simulink model "AA136_Sim"  (R2023b)
settings: Solver=VariableStepAuto  StartTime=0.0  StopTime=500  RelTol=1e-3
libraries: raspberrypiBasiclib x6
settings Model: Creator=ANWILEY-GREEN  LastModifiedBy=reedv

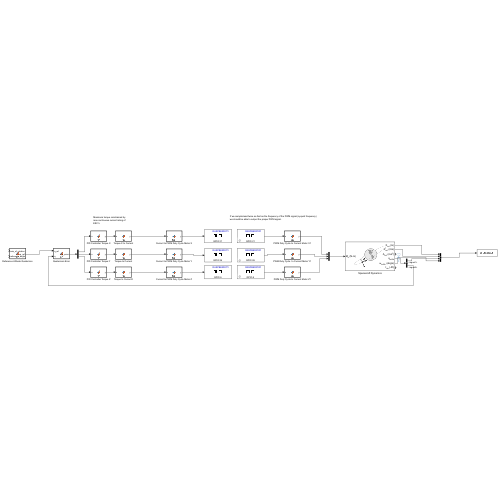
[thumbnail: Simulink's stored preview of the top-level diagram]
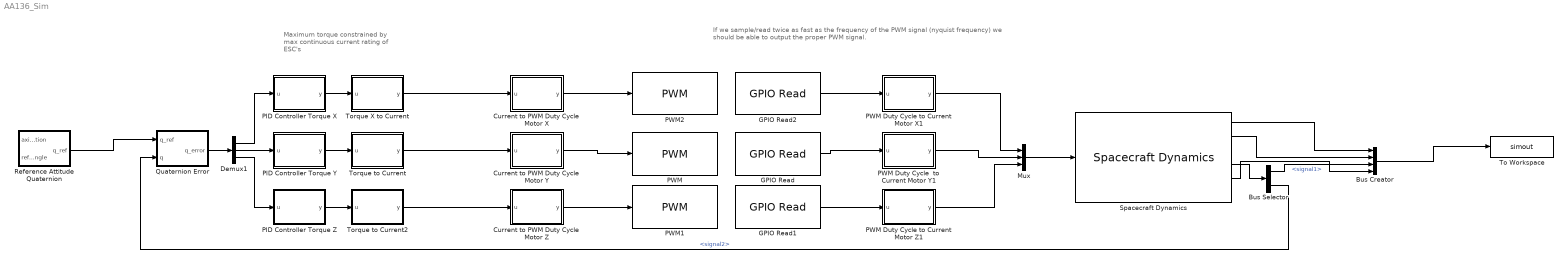
== system AA136_Sim ==
  note: Maximum torque constrained by
      | max continuous current rating of
      | ESC's
  note: If we sample/read twice as fast as the frequency of the PWM signal (nyquist frequency)
      | we should be able to output the proper PWM signal.
  Bus Creator : BusCreator  Inputs=4
  Bus Selector : BusSelector  OutputSignals=signal1,signal2
  Current to PWM Duty Cycle Motor X : MATLAB Function  TreatAsAtomicUnit=on
  Current to PWM Duty Cycle Motor Y : MATLAB Function  TreatAsAtomicUnit=on
  Current to PWM Duty Cycle Motor Z : MATLAB Function  TreatAsAtomicUnit=on
  Demux1 : Demux  Outputs=3
  GPIO Read : raspberrypiBasiclib/GPIO Read  board=Pi 4 Model B  gpio=26  internalResistor=Off  sampleTime=0.1  direction=Input  blockPlatform=Raspberry Pi
  GPIO Read1 : raspberrypiBasiclib/GPIO Read  board=Pi 4 Model B  gpio=6  internalResistor=Off  sampleTime=0.1  direction=Input  blockPlatform=Raspberry Pi
  GPIO Read2 : raspberrypiBasiclib/GPIO Read  board=Pi 4 Model B  gpio=21  internalResistor=Off  sampleTime=0.1  direction=Input  blockPlatform=Raspberry Pi
  Mux : Mux  Inputs=3
  PID Controller Torque X : MATLAB Function  TreatAsAtomicUnit=on
  PID Controller Torque Y : MATLAB Function  TreatAsAtomicUnit=on
  PID Controller Torque Z : MATLAB Function  TreatAsAtomicUnit=on
  PWM : raspberrypiBasiclib/PWM  board=Pi 2 Model B  Pin_=26  Frequency=50  blockPlatform=Raspberry Pi
  PWM Duty Cycle  to Current Motor Y1 : MATLAB Function  TreatAsAtomicUnit=on
  PWM Duty Cycle to Current Motor X1 : MATLAB Function  TreatAsAtomicUnit=on
  PWM Duty Cycle to Current Motor Z1 : MATLAB Function  TreatAsAtomicUnit=on
  PWM1 : raspberrypiBasiclib/PWM  board=Pi 2 Model B  Pin_=6  Frequency=50  blockPlatform=Raspberry Pi
  PWM2 : raspberrypiBasiclib/PWM  board=Pi 2 Model B  Pin_=21  Frequency=50  blockPlatform=Raspberry Pi
  Quaternion Error : MATLAB Function  TreatAsAtomicUnit=on
  Reference Attitude Quaternion : MATLAB Function  TreatAsAtomicUnit=on
  Spacecraft Dynamics : SpacecraftDynamics  forcesIn=off  outputAccel=on  attitudeRate=[1, 0, 0]  useDrag=on  MagneticIndexExtrapMethod=IGRF
  To Workspace : ToWorkspace  VariableName=simout  SaveFormat=Timeseries  SampleTime=-1
  Torque X to Current : MATLAB Function  TreatAsAtomicUnit=on
  Torque to Current : MATLAB Function  TreatAsAtomicUnit=on
  Torque to Current2 : MATLAB Function  TreatAsAtomicUnit=on
  wires:
  Spacecraft Dynamics/5 -> Bus Creator/4
  Spacecraft Dynamics/4 -> Bus Selector/1
  Bus Creator/1 -> To Workspace/1
  Spacecraft Dynamics/2 -> Bus Creator/2
  Spacecraft Dynamics/1 -> Bus Creator/1
  Reference Attitude Quaternion/1(q_ref) -> Quaternion Error/1(q_ref)
  Quaternion Error/1(q_error) -> Demux1/1
  PID Controller Torque Y/1(y) -> Torque to Current/1(u)
  Current to PWM Duty Cycle Motor Y/1(y) -> PWM/1
  Current to PWM Duty Cycle Motor X/1(y) -> PWM2/1
  Current to PWM Duty Cycle Motor Z/1(y) -> PWM1/1
  Demux1/1 -> PID Controller Torque X/1(u)
  Demux1/2 -> PID Controller Torque Y/1(u)
  Demux1/3 -> PID Controller Torque Z/1(u)
  PID Controller Torque X/1(y) -> Torque X to Current/1(u)
  PID Controller Torque Z/1(y) -> Torque to Current2/1(u)
  Torque X to Current/1(y) -> Current to PWM Duty Cycle Motor X/1(u)
  Torque to Current/1(y) -> Current to PWM Duty Cycle Motor Y/1(u)
  Torque to Current2/1(y) -> Current to PWM Duty Cycle Motor Z/1(u)
  Bus Selector/1 -> Bus Creator/3  "<signal1>"
  Bus Selector/2 -> Quaternion Error/2(q)  "<signal2>"
  PWM Duty Cycle to Current Motor X1/1(y) -> Mux/1
  PWM Duty Cycle to Current Motor Z1/1(y) -> Mux/3
  PWM Duty Cycle  to Current Motor Y1/1(y) -> Mux/2
  GPIO Read2/1 -> PWM Duty Cycle to Current Motor X1/1(u)
  GPIO Read/1 -> PWM Duty Cycle  to Current Motor Y1/1(u)
  GPIO Read1/1 -> PWM Duty Cycle to Current Motor Z1/1(u)
  Mux/1 -> Spacecraft Dynamics/1

== matlab function AA136_Sim/PWM Duty Cycle to Current Motor Z1 ==
  data: u input; y output
function y = fcn(u)

y = u;

== matlab function AA136_Sim/Reference Attitude Quaternion ==
  data: axis_of_rotation input; q_ref output; reference_angle input
function q_ref = fcn(axis_of_rotation, reference_angle)
    theta = deg2rad(reference_angle);
    q_ref = [cos(theta/2); axis_of_rotation*sin(theta/2)];
end

== matlab function AA136_Sim/PID Controller Torque Y ==
  data: u input; y output
function y = fcn(u)

y = u;

== matlab function AA136_Sim/Torque to Current ==
  data: u input; y output
function y = fcn(u)

y = u;

== matlab function AA136_Sim/Current to PWM Duty Cycle Motor Y ==
  data: u input; y output
function y = fcn(u)

y = u;

== matlab function AA136_Sim/Current to PWM Duty Cycle Motor X ==
  data: u input; y output
function y = fcn(u)

y = u;

== matlab function AA136_Sim/Current to PWM Duty Cycle Motor Z ==
  data: u input; y output
function y = fcn(u)

y = u;

== matlab function AA136_Sim/PID Controller Torque X ==
  data: u input; y output
function y = fcn(u)

y = u;

== matlab function AA136_Sim/PID Controller Torque Z ==
  data: u input; y output
function y = fcn(u)

y = u;

== matlab function AA136_Sim/Torque X to Current ==
  data: u input; y output
function y = fcn(u)

y = u;

== matlab function AA136_Sim/Quaternion Error ==
  data: q_ref input; q_error output; q input
function q_error = fcn(q_ref, q)
    q_c = quaternion_conjugate(q);
    q_err = multiply_quaternions(q_ref, q_c);
    angle_err = 2 * acos(q_error(1));
    axis_err = q_err(2:4) / norm(q_err(2:4));
    % Compute the error in the body frame
    q_error = angle_err * axis_err;
end
function q_prod = multiply_quaternions(q1, q2)
    % Quaternion multiplication
    a1 = q1(1);
    b1 = q1(2);
    c1 = q1(3);
    d1 = q1(4);

    a2 = q2(1);
    b2 = q2(2);
    c2 = q2(3);
    d2 = q2(4);

    q_prod = [a1*a2-b1*b2-c1*c2-d1*d2;
              a1*b2+b1*a2+c1*d2-d1*c2;
              a1*c2-b1*d2+c1*a2+d1*b2;
              a1*d2+b1*c2-c1*b2+d1*a2];
end

function q_conj = quaternion_conjugate(q)
    % Quaternion conjugate
    q_conj = [q(1); -q(2:4)];
end

== matlab function AA136_Sim/Torque to Current2 ==
  data: u input; y output
function y = fcn(u)

y = u;

== matlab function AA136_Sim/PWM Duty Cycle to Current Motor X1 ==
  data: u input; y output
function y = fcn(u)

y = u;

== matlab function AA136_Sim/PWM Duty Cycle  to Current Motor Y1 ==
  data: u input; y output
function y = fcn(u)

y = u;
